simulink model "RangingEstimatorV3"  (R2020b)
settings: Solver=FixedStepDiscrete  StartTime=0.0  StopTime=0.6  FixedStep=0.000001  RelTol=1e-3
settings Model: SILPILModeSetting=veronly  NumberOfSteps=1000  EnablePacing=on  ExtModeTrigDuration=2  Creator=拾夕  LastModifiedBy=拾夕
settings DataIOCC: SaveOutput=off  SaveTime=off
settings OptimizationCC: DefaultParameterBehavior=Inlined  EnhancedBackFolding=on  PassReuseOutputArgsAs=Individual arguments  MaxStackSize=64  OptimizeBlockOrder=speed  DifferentSizesBufferReuse=on  OptimizationCustomize=off  EfficientTunableParamExpr=on
settings DebuggingCC: ParameterTunabilityLossMsg=error
settings HardwareCC: ProdBitPerPointer=32  ProdBitPerSizeT=32  ProdBitPerPtrDiffT=32  ProdLargestAtomicInteger=Long  ProdLargestAtomicFloat=Double  ProdWordSize=32  ProdHWDeviceType=ARM Compatible->ARM Cortex-M
settings SFSimCC: MATLABDynamicMemAlloc=off
settings RTWCC: Description=Embedded Coder  SystemTargetFile=ert.tlc  GenCodeOnly=on  TemplateMakefile=ert_default_tmf  GenerateReport=on  RetainRTWFile=on  Toolchain=Arduino ARM  BuildConfiguration=Faster Runs  IncludeHyperlinkInReport=on  LaunchReport=on  GenerateWebview=on  GenerateCodeMetricsReport=on
settings CodeAppCC: ForceParamTrailComments=on  IgnoreCustomStorageClasses=off  OperatorAnnotations=on  SimulinkDataObjDesc=on  SFDataObjDesc=on  InsertBlockDesc=on
settings ERTTargetCC: CodeInterfacePackaging=Reusable function  SupportContinuousTime=on  ExtModeStaticAllocSize=250  ERTCustomFileTemplate=example_file_process.tlc  ERTFilePackagingFormat=Compact
settings ConfigComp: CovScope=Subsystem  CovHTMLOptions=-sRT=1 -sVT=1 -aTS=1 -agT=1 -bRG=1 -bTC=1 -hTR=0 -nFC=0 -nFD=1 -scm=1 -bcm=1 -xEv=0 -xEM=0 -req=1  CovSaveSingleToWorkspaceVar=on  CovExternalEMLEnable=off  CovSFcnEnable=off

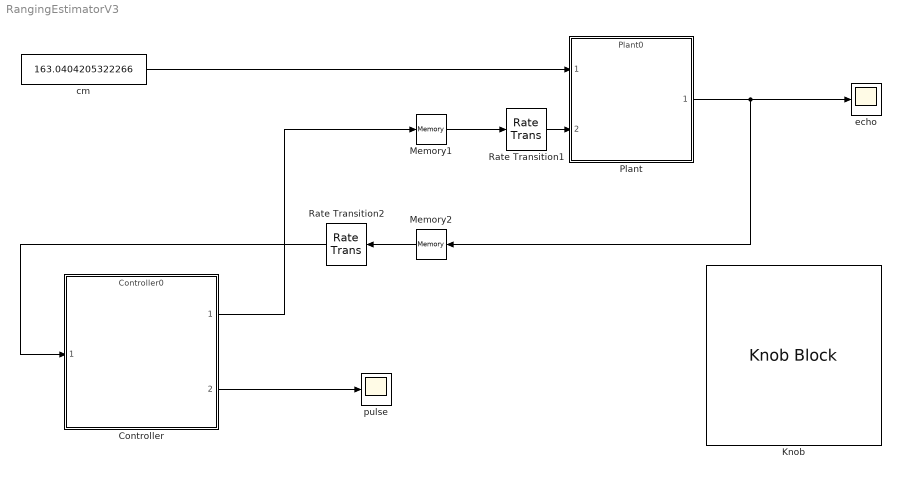
== system RangingEstimatorV3 ==
  Controller : ModelReference  ModelNameDialog=Controller0  SimulationMode=Normal  ModelReferenceVersion=1.25
  Knob : KnobBlock  ScaleMax=600
  Memory1 : Memory
  Memory2 : Memory
  Plant : ModelReference  ModelNameDialog=Plant0  SimulationMode=Normal  ModelReferenceVersion=1.23
  Rate Transition1 : RateTransition
  Rate Transition2 : RateTransition
  cm : Constant  Value=163.0404205322266  OutDataTypeStr=single
  echo : Scope
  pulse : Scope
  wires:
  cm/1 -> Plant/1
  Memory1/1 -> Rate Transition1/1
  Rate Transition1/1 -> Plant/2
  Plant/1 -> Memory2/1, echo/1
  Controller/1 -> Memory1/1
  Controller/2 -> pulse/1
  Memory2/1 -> Rate Transition2/1
  Rate Transition2/1 -> Controller/1
